simulink model "Electromech_sys_nonlinear_obs"  (R2025b)
settings: Solver=ode15s  StartTime=0.0  StopTime=12  RelTol=1e-3
values from neighbouring files (symbols this model uses):
  p_0 = 0    [Init_Simulink_param_nl_Electromech.m]
  phat_0 = 1e-3    (= 0.001)    [Init_Simulink_param_nl_Electromech.m]
  q_0 = 0    [Init_Simulink_param_nl_Electromech.m]
  Q_0 = 0    [Init_Simulink_param_nl_Electromech.m]
  qhat_0 = 2e-4    (= 0.0002)    [Init_Simulink_param_nl_Electromech.m]
  Qhat_0 = 5e-8    (= 5e-08)    [Init_Simulink_param_nl_Electromech.m]
undefined symbols (not defined in the file or in its folder): params
settings Model: Creator=filippougolini  LastModifiedBy=filippougolini

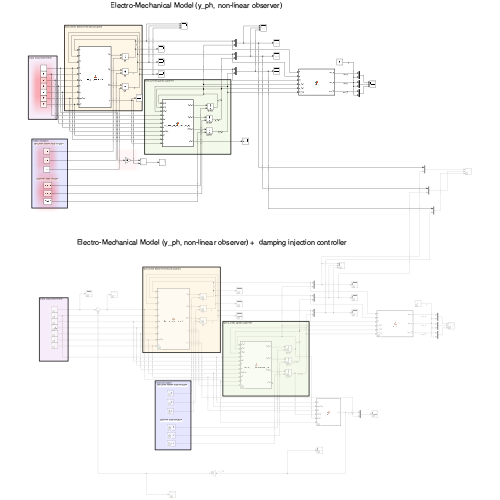
[thumbnail: Simulink's stored preview of the top-level diagram]
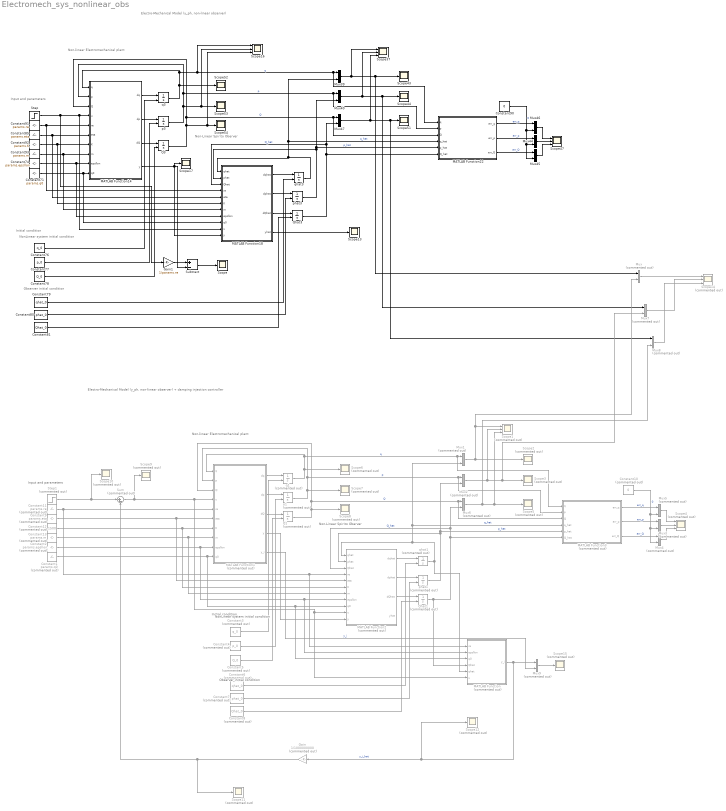
== system Electromech_sys_nonlinear_obs ==
  note: Initial condition
  note: Non-Linear Spirito Oberver
  note: Input and parameters
  note: NonLinear system initial condition
  note: Observer initial condition
  note: Electro-Mechanical Model (y_ph, non-linear observer)
  note: Non-linear Electromechanical plant
  note: Observer initial condition
  note: Non-Linear Spirito Oberver
  note: Initial condition
  note: NonLinear system initial condition
  note: Non-linear Electromechanical plant
  note: Input and parameters
  note: Electro-Mechanical Model (y_ph, non-linear observer) + damping injection controller
  Constant1 : Constant  Commented=on  Value=params.q0
  Constant10 : Constant  Commented=on  Value=0
  Constant11 : Constant  Commented=on  Value=params.re
  Constant12 : Constant  Commented=on  Value=1500
  Constant13 : Constant  Commented=on  Value=params.m
  Constant2 : Constant  Commented=on  Value=params.epsllon
  Constant3 : Constant  Commented=on  Value=q_0
  Constant4 : Constant  Commented=on  Value=p_0
  Constant5 : Constant  Commented=on  Value=Q_0
  Constant6 : Constant  Commented=on  Value=qhat_0
  Constant7 : Constant  Commented=on  Value=phat_0
  Constant71 : Constant  Value=params.q0
  Constant74 : Constant  Value=params.epsllon
  Constant76 : Constant  Value=q_0
  Constant77 : Constant  Value=p_0
  Constant78 : Constant  Value=Q_0
  Constant79 : Constant  Value=qhat_0
  Constant8 : Constant  Commented=on  Value=Qhat_0
  Constant80 : Constant  Value=phat_0
  Constant81 : Constant  Value=Qhat_0
  Constant85 : Constant  Value=params.eta
  Constant9 : Constant  Commented=on  Value=params.eta
  Constant90 : Constant  Value=0
  Constant91 : Constant  Value=params.re
  Constant92 : Constant  Value=params.K
  Constant93 : Constant  Value=params.m
  Gain : Gain  Commented=on  Gain=1/1000000000
  Gain1 : Gain  Gain=1/params.re
  MATLAB Function : MATLAB Function  Commented=on  TreatAsAtomicUnit=on
  MATLAB Function1 : MATLAB Function  Commented=on  TreatAsAtomicUnit=on
  MATLAB Function14 : MATLAB Function  TreatAsAtomicUnit=on
  MATLAB Function18 : MATLAB Function  TreatAsAtomicUnit=on
  MATLAB Function2 : MATLAB Function  Commented=on  TreatAsAtomicUnit=on
  MATLAB Function22 : MATLAB Function  TreatAsAtomicUnit=on
  MATLAB Function3 : MATLAB Function  Commented=on  TreatAsAtomicUnit=on
  Mux{,1..9} (10 alike) : Mux  Commented=on  Inputs=2
  Mux{39..40,44..47} (6 alike) : Mux  Inputs=2
  Q1 : Integrator  Commented=on  InitialConditionSource=external
  Q3 : Integrator  InitialConditionSource=external
  Qhat1 : Integrator  Commented=on  InitialConditionSource=external  InitialCondition=30e-9
  Qhat3 : Integrator  InitialConditionSource=external  InitialCondition=30e-9
  Scope{,13,17,43..44,51..54} (9 alike) : Scope
      Scope settings: ActiveDisplayYMinimum=-136.48775967186276  ActiveDisplayYMaximum=1157.3875288524291  DataLoggingVariableName=ScopeData17
      Scope13 settings: ActiveDisplayYMinimum=-388.73037301174418  ActiveDisplayYMaximum=1956.89498755588  DataLoggingVariableName=ScopeData12
      Scope17 settings: ActiveDisplayYMinimum=-149.59459313180929  ActiveDisplayYMaximum=1346.3513381862838  DataLoggingVariableName=ScopeData16
      Scope43 settings: ActiveDisplayYMinimum=-4.4929456410290065E-5  ActiveDisplayYMaximum=0.00036894675529116814  DataLoggingVariableName=ScopeData43
      Scope44 settings: ActiveDisplayYMinimum=-1  ActiveDisplayYMaximum=1  DataLoggingVariableName=ScopeData44
      Scope51 settings: ActiveDisplayYMinimum=-1  ActiveDisplayYMaximum=1  DataLoggingVariableName=ScopeData51
      Scope52 settings: ActiveDisplayYMinimum=-4.0944874698701246E-5  ActiveDisplayYMaximum=0.0003685038722883113  DataLoggingVariableName=ScopeData52
      Scope53 settings: ActiveDisplayYMinimum=-1  ActiveDisplayYMaximum=1  DataLoggingVariableName=ScopeData53
      Scope54 settings: ActiveDisplayYMinimum=-1  ActiveDisplayYMaximum=1  DataLoggingVariableName=ScopeData54
  Scope1 : Scope  Commented=on  NumInputPorts=3
      settings: ActiveDisplayYMinimum=-2.573333017477019E-5  ActiveDisplayYMaximum=0.00022790522393242347
  Scope{2..3,5..12,15} (11 alike) : Scope  Commented=on
      Scope10 settings: ActiveDisplayYMinimum=4999.9999970462986  ActiveDisplayYMaximum=5000.0000028194981  DataLoggingVariableName=ScopeData9
      Scope11 settings: ActiveDisplayYMinimum=-113.45438996779558  ActiveDisplayYMaximum=649.107422097647  DataLoggingVariableName=ScopeData10
      Scope12 settings: ActiveDisplayYMinimum=-0.582081690905234  ActiveDisplayYMaximum=4.5825804840759048  DataLoggingVariableName=ScopeData11
      Scope15 settings: ActiveDisplayYMinimum=-2033.5568970200575  ActiveDisplayYMaximum=1113.0654514328378  DataLoggingVariableName=ScopeData14
      Scope2 settings: ActiveDisplayYMinimum=-4.4929456410290065E-5  ActiveDisplayYMaximum=0.00036894675529116814
      Scope3 settings: ActiveDisplayYMinimum=-1  ActiveDisplayYMaximum=1  DataLoggingVariableName=ScopeData2
      Scope5 settings: ActiveDisplayYMinimum=-1  ActiveDisplayYMaximum=1  DataLoggingVariableName=ScopeData4
      Scope6 settings: ActiveDisplayYMinimum=-4.0944874698701246E-5  ActiveDisplayYMaximum=0.0003685038722883113  DataLoggingVariableName=ScopeData5
      Scope7 settings: ActiveDisplayYMinimum=-1  ActiveDisplayYMaximum=1  DataLoggingVariableName=ScopeData6
      Scope8 settings: ActiveDisplayYMinimum=-1  ActiveDisplayYMaximum=1  DataLoggingVariableName=ScopeData7
      Scope9 settings: ActiveDisplayYMinimum=-1337.3007056129782  ActiveDisplayYMaximum=9705.1568768429333  DataLoggingVariableName=ScopeData8
  Scope14 : Scope  Commented=on  NumInputPorts=3
      settings: ActiveDisplayYMinimum=-0.00010478939543296066  ActiveDisplayYMaximum=0.00023634749570294747  DataLoggingVariableName=ScopeData13
  Scope16 : Scope  NumInputPorts=3
      settings: ActiveDisplayYMinimum=-1  ActiveDisplayYMaximum=1  DataLoggingVariableName=ScopeData15
  Scope37 : Scope  NumInputPorts=3
      settings: ActiveDisplayString=3  ActiveDisplayYMinimum=-9.5553725594488087E-9  ActiveDisplayYMaximum=7.555901607850705E-8  DataLoggingVariableName=ScopeData37
  Scope4 : Scope  Commented=on  NumInputPorts=3
      settings: ActiveDisplayYMinimum=-0.0014645136103350045  ActiveDisplayYMaximum=0.003180620537022315  DataLoggingVariableName=ScopeData3
  Scope47 : Scope  NumInputPorts=3
      settings: ActiveDisplayYMinimum=-0.0014645136103350045  ActiveDisplayYMaximum=0.003180620537022315  DataLoggingVariableName=ScopeData47
  Step : Step  After=5140  SampleTime=0
  Step1 : Step  Commented=on  After=4e3  SampleTime=0
  Subtract : Sum  Inputs=+-
  Sum : Sum  Commented=on  Inputs=|+-
  p1 : Integrator  Commented=on  InitialConditionSource=external
  p3 : Integrator  InitialConditionSource=external
  phat1 : Integrator  Commented=on  InitialConditionSource=external  InitialCondition=5e-4
  phat3 : Integrator  InitialConditionSource=external  InitialCondition=5e-4
  q1 : Integrator  Commented=on  InitialConditionSource=external
  q3 : Integrator  InitialConditionSource=external
  qhat1 : Integrator  Commented=on  InitialConditionSource=external  InitialCondition=20e-5
  qhat3 : Integrator  InitialConditionSource=external  InitialCondition=20e-5
  wires:
  Constant79/1 -> qhat3/2
  MATLAB Function14/2(dp) -> p3/1
  Constant92/1 -> MATLAB Function14/7(K), MATLAB Function18/6(K)
  Constant91/1 -> MATLAB Function14/5(re), MATLAB Function18/4(re)
  Constant74/1 -> MATLAB Function14/9(epsllon), MATLAB Function18/8(epsllon)
  Constant85/1 -> MATLAB Function14/6(eta), MATLAB Function18/5(eta)
  Constant76/1 -> q3/2
  phat3/1 -> MATLAB Function22/5(p_hat), Mux40/2, MATLAB Function18/2(phat)  "p_hat"
  MATLAB Function14/4(y) -> Subtract/2, Scope17/1, MATLAB Function18/11(y)
  p3/1 -> Scope16/2, Scope53/1, Mux40/1, MATLAB Function22/2(p), MATLAB Function14/2(p)  "p"
  qhat3/1 -> Mux39/2, MATLAB Function22/4(q_hat), MATLAB Function18/1(qhat)  "q_hat"
  Constant93/1 -> MATLAB Function14/8(m), MATLAB Function18/7(m)
  Mux45/1 -> Scope47/3
  Constant78/1 -> Q3/2
  MATLAB Function18/1(dqhat) -> qhat3/1
  Step/1 -> Gain1/1, MATLAB Function18/10(u), MATLAB Function14/4(u)
  Q3/1 -> Mux47/1, MATLAB Function22/3(Q), MATLAB Function14/3(Q), Scope16/3, Scope54/1  "Q"
  Mux40/1 -> Scope37/2, Mux7/1, Scope44/1
  MATLAB Function22/1(err_q) -> Mux46/1  "err_q"
  Constant80/1 -> phat3/2
  MATLAB Function18/2(dphat) -> phat3/1
  Constant71/1 -> MATLAB Function18/9(q0), MATLAB Function14/10(q0)
  Mux47/1 -> Scope37/3, Mux8/1, Scope51/1
  Mux39/1 -> Scope37/1, Scope43/1, Mux/1
  Mux46/1 -> Scope47/1
  Constant81/1 -> Qhat3/2
  Constant90/1 -> Mux45/2, Mux44/2, Mux46/2  "0"
  Qhat3/1 -> MATLAB Function22/6(Q_hat), Mux47/2, MATLAB Function18/3(Qhat)  "Q_hat"
  MATLAB Function18/3(dQhat) -> Qhat3/1
  MATLAB Function14/3(dQ) -> Q3/1
  MATLAB Function14/1(dq) -> q3/1
  q3/1 -> Scope52/1, MATLAB Function14/1(q), Scope16/1, Mux39/1, MATLAB Function22/1(q)  "q"
  Constant77/1 -> p3/2
  MATLAB Function22/3(err_Q) -> Mux45/1  "err_Q"
  MATLAB Function22/2(err_p) -> Mux44/1  "err_p"
  Mux44/1 -> Scope47/2
  Mux4/1 -> Scope4/3
  Sum/1 -> MATLAB Function/6(u), MATLAB Function2/10(u), MATLAB Function1/4(u), Scope9/1
  Mux5/1 -> Scope4/1
  Constant10/1 -> Mux4/2, Mux3/2, Mux5/2  "0"
  MATLAB Function2/2(dphat) -> phat1/1
  MATLAB Function3/3(err_Q) -> Mux4/1  "err_Q"
  MATLAB Function1/3(dQ) -> Q1/1
  qhat1/1 -> Mux1/2, MATLAB Function3/4(q_hat), MATLAB Function2/1(qhat), MATLAB Function/5(qhat)  "q_hat"
  MATLAB Function1/2(dp) -> p1/1
  Constant7/1 -> phat1/2
  Mux1/1 -> Scope1/1, Mux/2, Scope2/1
  MATLAB Function3/2(err_p) -> Mux3/1  "err_p"
  MATLAB Function2/1(dqhat) -> qhat1/1
  Constant1/1 -> MATLAB Function/3(q0), MATLAB Function2/9(q0), MATLAB Function1/10(q0)
  Mux2/1 -> Scope1/2, Scope3/1, Mux7/2
  Constant2/1 -> MATLAB Function1/9(epsllon), MATLAB Function/2(epsllon), MATLAB Function2/8(epsllon)
  phat1/1 -> MATLAB Function3/5(p_hat), Mux2/2, MATLAB Function2/2(phat)  "p_hat"
  q1/1 -> Scope6/1, MATLAB Function1/1(q), Mux1/1, MATLAB Function3/1(q)  "q"
  MATLAB Function2/3(dQhat) -> Qhat1/1
  Constant8/1 -> Qhat1/2
  Mux6/1 -> Scope5/1, Scope1/3, Mux8/2
  Qhat1/1 -> MATLAB Function/4(Qhat), MATLAB Function3/6(Q_hat), Mux6/2, MATLAB Function2/3(Qhat)  "Q_hat"
  p1/1 -> Scope7/1, Mux2/1, MATLAB Function3/2(p), MATLAB Function1/2(p)  "p"
  Constant3/1 -> q1/2
  MATLAB Function1/1(dq) -> q1/1
  Constant5/1 -> Q1/2
  MATLAB Function3/1(err_q) -> Mux5/1  "err_q"
  Q1/1 -> Mux6/1, MATLAB Function3/3(Q), MATLAB Function1/3(Q), Scope8/1  "Q"
  Constant11/1 -> MATLAB Function1/5(re), MATLAB Function/1(re), MATLAB Function2/4(re)
  Constant6/1 -> qhat1/2
  Constant13/1 -> MATLAB Function1/8(m), MATLAB Function2/7(m)
  Mux3/1 -> Scope4/2
  MATLAB Function1/4(y) -> MATLAB Function2/11(y)
  Constant4/1 -> p1/2
  Constant9/1 -> MATLAB Function1/6(eta), MATLAB Function2/5(eta)
  Constant12/1 -> MATLAB Function1/7(K), MATLAB Function2/6(K)
  Step1/1 -> Sum/1, Scope10/1
  Gain/1 -> Sum/2, Scope11/1
  MATLAB Function18/4(yhat) -> Scope13/1
  MATLAB Function/1(y_i) -> Mux9/1, Scope12/1, Gain/1  "y_i_hat"
  Mux/1 -> Scope14/1
  Mux7/1 -> Scope14/2
  Mux8/1 -> Scope14/3
  MATLAB Function1/5(y_i) -> Mux9/2  "y_i"
  Mux9/1 -> Scope15/1
  Gain1/1 -> Subtract/1
  Subtract/1 -> Scope/1

== matlab function Electromech_sys_nonlinear_obs/MATLAB Function18 ==
  data: qhat input; phat input; Qhat input; re input; eta input; K input; m input; epsllon input; q0 input; u input; dqhat output; y input; dphat output; dQhat output; yhat output
function [dqhat, dphat, dQhat, yhat] = observer_pH_electromech_yph(qhat, phat, Qhat, ...
    re, eta, K, m, epsllon, q0, u, y)

    % Port-Hamiltonian structure matrices
    J = [  0  1  0;
          -1  0  0;
           0  0  0 ];

    R = diag([0, eta, 1/re]);
    g = [0; 0; 1/re];

    % -------- Hamiltonian gradient at xhat = [qhat; phat; Qhat] --------
    Cqh    = epsllon * (qhat + q0)^4;

    % dH/dqhat
    dHhdqh = K*qhat - 2*Qhat^2 / (epsllon * (qhat + q0)^5);
    % dH/dphat
    dHhdph = phat / m;
    % dH/dQhat
    dHhdQh = Qhat / Cqh;

    gradHh = [dHhdqh; dHhdph; dHhdQh];
    
    % -------- Observer gain L --------
    gamma = 20;
    L  = gamma * g;
    Lcol = L.';       % ensure it's 3x1

    yhat = Qhat / (re * epsllon * (qhat + q0)^4);

    % -------- Observer dynamics --------
    % Note: J and R are constant
    xhatdot = (J - R) * gradHh + g*u + Lcol * (y - yhat);

    dqhat = xhatdot(1);
    dphat = xhatdot(2);
    dQhat = xhatdot(3);
end

== matlab function Electromech_sys_nonlinear_obs/MATLAB Function22 ==
  data: q input; err_q output; p input; Q input; q_hat input; p_hat input; Q_hat input; err_p output; err_Q output
function [err_q, err_p, err_Q] = error(q, p, Q, q_hat, p_hat, Q_hat)

    err_q = q - q_hat;
    err_p = p - p_hat;
    err_Q = Q - Q_hat;
end

== matlab function Electromech_sys_nonlinear_obs/MATLAB Function1 ==
  data: q input; p input; Q input; u input; dq output; re input; eta input; K input; m input; epsllon input; q0 input; dp output; dQ output; y output; y_i output
function [dq, dp, dQ, y, y_i] = plant_pH_electromech(q, p, Q, u, re, eta, K, m, epsllon, q0)
% Electro-mechanical pH plant

    % Parameters: m, K, eta, eps, re, q0 in workspace

    J = [  0  1  0;
          -1  0  0;
           0  0  0 ];

    R = diag([0, eta, 1/re]);
    g = [0; 0; 1/re];

    % Hamiltonian gradient gradH(q,p,Q)
    Cq   = epsllon * (q + q0)^4;

    dHdq = K*q - 2*Q^2 / (epsllon * (q + q0)^5);
    dHdp = p / m;
    dHdQ = Q / Cq;

    gradH = [dHdq; dHdp; dHdQ];

    xdot = (J - R) * gradH + g*u;

    y = Q / (re * epsllon * (q + q0)^4);
    y_i = - Q / (re * epsllon * (q + q0)^4) + u/re;


    
    dq = xdot(1);
    dp = xdot(2);
    dQ = xdot(3);
end

== matlab function Electromech_sys_nonlinear_obs/MATLAB Function2 ==
  data: qhat input; phat input; Qhat input; re input; eta input; K input; m input; epsllon input; q0 input; u input; dqhat output; y input; dphat output; dQhat output; yhat output
function [dqhat, dphat, dQhat, yhat] = observer_pH_electromech_yph(qhat, phat, Qhat, ...
    re, eta, K, m, epsllon, q0, u, y)

    % Port-Hamiltonian structure matrices
    J = [  0  1  0;
          -1  0  0;
           0  0  0 ];

    R = diag([0, eta, 1/re]);
    g = [0; 0; 1/re];

    % -------- Hamiltonian gradient at xhat = [qhat; phat; Qhat] --------
    Cqh    = epsllon * (qhat + q0)^4;

    % dH/dqhat
    dHhdqh = K*qhat - 2*Qhat^2 / (epsllon * (qhat + q0)^5);
    % dH/dphat
    dHhdph = phat / m;
    % dH/dQhat
    dHhdQh = Qhat / Cqh;

    gradHh = [dHhdqh; dHhdph; dHhdQh];
    
    % -------- Observer gain L --------
    gamma = 20;
    L  = gamma * g;
    Lcol = L.';       % ensure it's 3x1

    yhat = Qhat / (re * epsllon * (qhat + q0)^4);
    y_i = - Qhat / (re * epsllon * (qhat + q0)^4) + u/re;

    % -------- Observer dynamics --------
    % Note: J and R are constant
    xhatdot = (J - R) * gradHh + g*u + Lcol * (y - yhat);

    dqhat = xhatdot(1);
    dphat = xhatdot(2);
    dQhat = xhatdot(3);
end

== matlab function Electromech_sys_nonlinear_obs/MATLAB Function3 ==
  data: q input; err_q output; p input; Q input; q_hat input; p_hat input; Q_hat input; err_p output; err_Q output
function [err_q, err_p, err_Q] = error(q, p, Q, q_hat, p_hat, Q_hat)

    err_q = q - q_hat;
    err_p = p - p_hat;
    err_Q = Q - Q_hat;
end

== matlab function Electromech_sys_nonlinear_obs/MATLAB Function ==
  data: re input; y_i output; epsllon input; q0 input; Qhat input; qhat input; u input
function y_i = fcn(re, epsllon, q0, Qhat, qhat, u)

y_i = - Qhat / (re * epsllon * (qhat + q0)^4) + u/re;
end

== matlab function Electromech_sys_nonlinear_obs/MATLAB Function14 ==
  data: q input; p input; Q input; u input; dq output; re input; eta input; K input; m input; epsllon input; q0 input; dp output; dQ output; y output
function [dq, dp, dQ, y] = plant_pH_electromech(q, p, Q, u, re, eta, K, m, epsllon, q0)
% Electro-mechanical pH plant

    % Parameters: m, K, eta, eps, re, q0 in workspace

    J = [  0  1  0;
          -1  0  0;
           0  0  0 ];

    R = diag([0, eta, 1/re]);
    g = [0; 0; 1/re];

    % Hamiltonian gradient gradH(q,p,Q)
    Cq   = epsllon * (q + q0)^4;

    dHdq = K*q - 2*Q^2 / (epsllon * (q + q0)^5);
    dHdp = p / m;
    dHdQ = Q / Cq;

    gradH = [dHdq; dHdp; dHdQ];

    xdot = (J - R) * gradH + g*u;

    y = Q / (re * epsllon * (q + q0)^4);

    
    dq = xdot(1);
    dp = xdot(2);
    dQ = xdot(3);
end
